simulink model "threeDiskOscillatorRig"  (R2024a)
settings: Solver=VariableStepAuto  StartTime=0.0  StopTime=SIM_TIME  RelTol=1e-8
values from neighbouring files (symbols this model uses):
  C = [0 0 0 0 1 0]    [Assignment2.m]
undefined symbols (not defined in the file or in its folder): atan_scale, b_1, b_2, b_3, J_1, J_2, J_3, k_1, k_2, Kred_tf_d, sigma1, SIM_TIME, T_Cm, T_Cp, T_s, w_th, x_0
libraries: simulink x1
settings Model: Creator=dimpa  LastModifiedBy=szica
settings SolverCC: AlgebraicLoopSolver=TrustRegion
settings DataIOCC: ReturnWorkspaceOutputs=off
settings DebuggingCC: UnconnectedInputMsg=warning  UnconnectedOutputMsg=warning  UnconnectedLineMsg=warning  ArithmeticOperatorsInVariantConditions=warning
settings ModelReferenceCC: EnableRefExpFcnMdlSchedulingChecks=on
settings SFSimCC: SimUseLocalCustomCode=off  CustomCodeUndefinedFunction=UseInterfaceOnly
settings RTWCC: RTWUseLocalCustomCode=off  GPUComputeCapability=3.5  DLArmComputeVersion=19.05

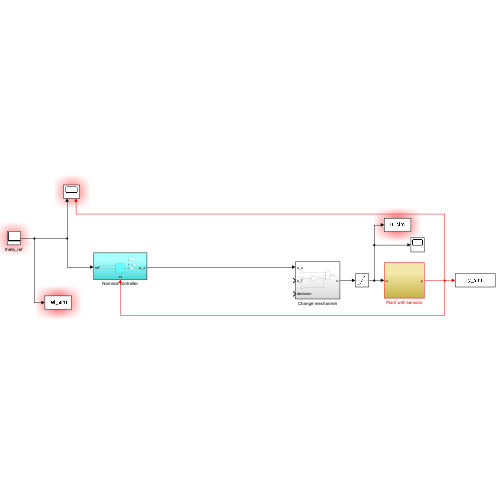
[thumbnail: Simulink's stored preview of the top-level diagram]
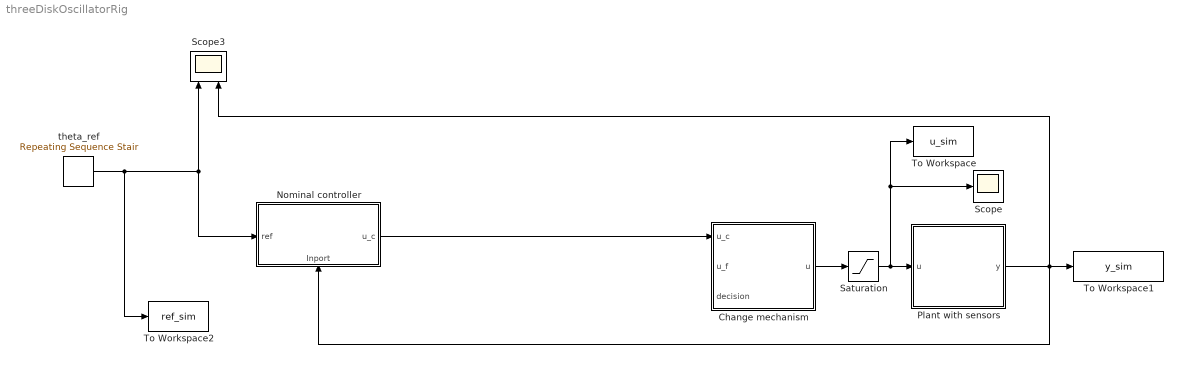
== system threeDiskOscillatorRig ==
  Change mechanism : Subsystem
  Nominal controller : Subsystem
      settings: PortSchema="{\"entries\":[{\"content\":{\"sides\":[{\"content\":{\"connectorIds\":[\"In1\"]},\"type\":\"ConnectorPlacement.EquallySpacedRectSide\",\"uuid\":\"4a12b61f-9c5c-4b70-9adc-3d80c48385d1\"},{\"content\":{\"connectorIds\":[\"Out1\"],\"side\":\"RIGHT\"},\"type\":\"ConnectorPlacement.EquallySpacedRectSide\",\"uuid\":\"2083013e-02ec-4e33-92aa-a5e5c42c1a52\"},{\"content\":{\"side\":\"TOP\"},\"type\":\"ConnectorPlacement.EquallySpacedRectSide\",\"uuid\":\"64789157-88d0-4aa4-87ae-72576a40396a\"},{\"content\":{\"connectorIds\":[\"In2\"],\"side\":\"BOTTOM\"},\"type\":\"ConnectorPlacement.EquallySpacedRectSide\",\"uuid\":\"628a79db-f9b2-407d-a20c-25144858a4c1\"}]},\"type\":\"ConnectorPlacement.EquallySpacedConnector\",\"uuid\":\"5f7ce1a9-4de3-49cc-b1cc-2f956a8eb5ad\"}],\"packageUris\":[\"http://schema.mathworks.com/mf0/Connector/R2020b\"],\"version\":\"1.0\"}"
  Plant with sensors : Subsystem
  Saturation : Saturate  UpperLimit=2  LowerLimit=-2
  Scope : Scope
  Scope3 : Scope  NumInputPorts=2
  To Workspace : ToWorkspace  VariableName=u_sim  SaveFormat=Timeseries  SampleTime=T_s
  To Workspace1 : ToWorkspace  VariableName=y_sim  SaveFormat=Timeseries  SampleTime=-1
  To Workspace2 : ToWorkspace  VariableName=ref_sim  SaveFormat=Timeseries  SampleTime=T_s
  theta_ref : simulink/Sources/Repeating Sequence Stair  OutValues=[0 0 0]  tsamp=SIM_TIME/2  OutMin=[]  OutMax=[]  OutDataTypeStr=double  OutputDataTypeScalingMode=double  OutDataType=fixdt(0,8)  ConRadixGroup=Best Precision: Vector-wise  OutScaling=2^-12
  wires:
  Plant with sensors/1(y) -> To Workspace1/1, Scope3/2, Nominal controller/2(Inport)
  theta_ref/1 -> Nominal controller/1(ref), Scope3/1, To Workspace2/1
  Change mechanism/1(u) -> Saturation/1
  Nominal controller/1(u_c) -> Change mechanism/1(u_c)
  Saturation/1 -> To Workspace/1, Scope/1, Plant with sensors/1(u)

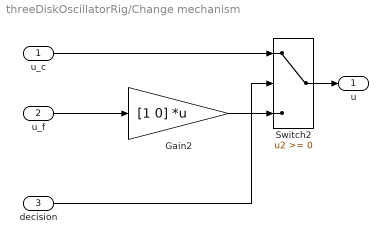
== system threeDiskOscillatorRig/Change mechanism ==
  u_c : Inport
  u_f : Inport  Port=2
  decision : Inport  Port=3
  Gain2 : Gain  Gain=[1 0]  Multiplication=Matrix(K*u) (u vector)
  Switch2 : Switch  OutDataTypeStr=double  SaturateOnIntegerOverflow=off  InputSameDT=off
  u : Outport
  wires:
  Gain2/1 -> Switch2/3
  decision/1 -> Switch2/2
  u_c/1 -> Switch2/1
  Switch2/1 -> u/1
  u_f/1 -> Gain2/1

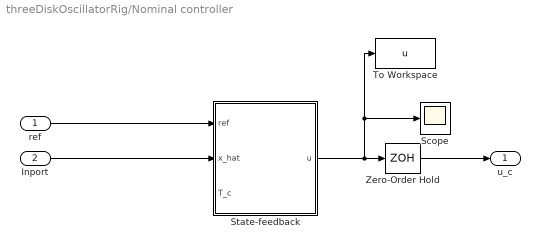
== system threeDiskOscillatorRig/Nominal controller ==
  ref : Inport
  Inport : Inport  Port=2
  Scope : Scope
  State-feedback : Subsystem
  To Workspace : ToWorkspace  VariableName=u  SaveFormat=Timeseries  SampleTime=T_s
  Zero-Order Hold : ZeroOrderHold  SampleTime=T_s
  u_c : Outport
  wires:
  Zero-Order Hold/1 -> u_c/1
  ref/1 -> State-feedback/1(ref)
  State-feedback/1(u) -> To Workspace/1, Scope/1, Zero-Order Hold/1
  Inport/1 -> State-feedback/2(x_hat)

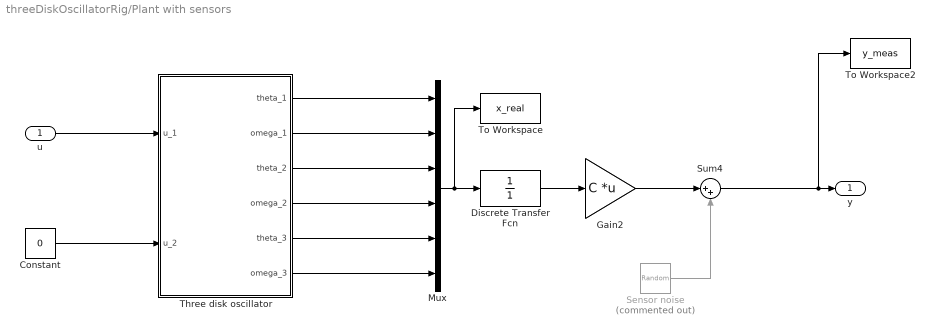
== system threeDiskOscillatorRig/Plant with sensors ==
  u : Inport
  Constant : Constant  Value=0
  Discrete Transfer Fcn : DiscreteTransferFcn  Denominator=[1]  SampleTime=T_s
  Gain2 : Gain  Gain=C  Multiplication=Matrix(K*u) (u vector)
  Mux : Mux  Inputs=6
  Sensor noise : RandomNumber  Commented=on  Variance=sigma1  SampleTime=T_s
  Sum4 : Sum  Inputs=|++
  Three disk oscillator : Subsystem
  To Workspace : ToWorkspace  VariableName=x_real  SaveFormat=Timeseries  SampleTime=T_s
  To Workspace2 : ToWorkspace  VariableName=y_meas  SaveFormat=Timeseries  SampleTime=T_s
  y : Outport  VectorParamsAs1DForOutWhenUnconnected=off
  wires:
  Three disk oscillator/2(omega_1) -> Mux/2
  Three disk oscillator/1(theta_1) -> Mux/1
  Mux/1 -> To Workspace/1, Discrete Transfer Fcn/1
  Three disk oscillator/4(omega_2) -> Mux/4
  Three disk oscillator/3(theta_2) -> Mux/3
  Discrete Transfer Fcn/1 -> Gain2/1
  Gain2/1 -> Sum4/1
  Sensor noise/1 -> Sum4/2
  Three disk oscillator/6(omega_3) -> Mux/6
  Three disk oscillator/5(theta_3) -> Mux/5
  Sum4/1 -> To Workspace2/1, y/1
  u/1 -> Three disk oscillator/1(u_1)
  Constant/1 -> Three disk oscillator/2(u_2)

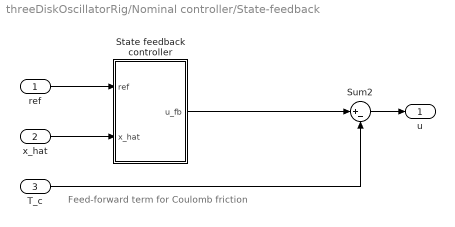
== system threeDiskOscillatorRig/Nominal controller/State-feedback ==
  note: Feed-forward term for Coulomb friction
  ref : Inport
  x_hat : Inport  Port=2
  T_c : Inport  Port=3
  State feedback controller : Subsystem
  Sum2 : Sum  Inputs=|+-
  u : Outport  VectorParamsAs1DForOutWhenUnconnected=off
  wires:
  T_c/1 -> Sum2/2
  Sum2/1 -> u/1
  ref/1 -> State feedback controller/1(ref)
  x_hat/1 -> State feedback controller/2(x_hat)
  State feedback controller/1(u_fb) -> Sum2/1

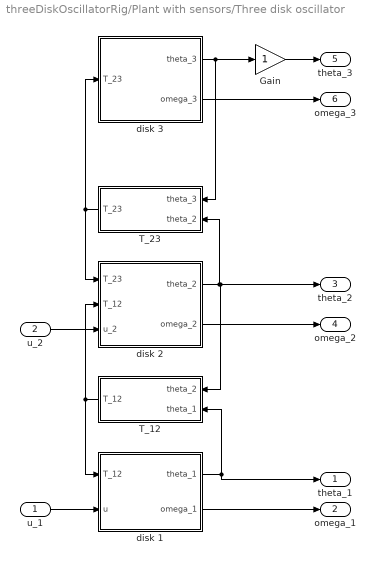
== system threeDiskOscillatorRig/Plant with sensors/Three disk oscillator ==
  u_1 : Inport
  u_2 : Inport  Port=2
  Gain : Gain
  T_12 : Subsystem
  T_23 : Subsystem
  disk 1 : Subsystem
  disk 2 : Subsystem
  disk 3 : Subsystem
  theta_1 : Outport  VectorParamsAs1DForOutWhenUnconnected=off
  omega_1 : Outport  Port=2  VectorParamsAs1DForOutWhenUnconnected=off
  theta_2 : Outport  Port=3  VectorParamsAs1DForOutWhenUnconnected=off
  omega_2 : Outport  Port=4  VectorParamsAs1DForOutWhenUnconnected=off
  theta_3 : Outport  Port=5  VectorParamsAs1DForOutWhenUnconnected=off
  omega_3 : Outport  Port=6  VectorParamsAs1DForOutWhenUnconnected=off
  wires:
  T_23/1(T_23) -> disk 2/1(T_23), disk 3/1(T_23)
  disk 1/1(theta_1) -> theta_1/1, T_12/2(theta_1)
  disk 2/1(theta_2) -> T_23/2(theta_2), theta_2/1, T_12/1(theta_2)
  T_12/1(T_12) -> disk 1/1(T_12), disk 2/2(T_12)
  disk 3/2(omega_3) -> omega_3/1
  disk 1/2(omega_1) -> omega_1/1
  disk 2/2(omega_2) -> omega_2/1
  u_1/1 -> disk 1/2(u)
  disk 3/1(theta_3) -> Gain/1, T_23/1(theta_3)
  Gain/1 -> theta_3/1
  u_2/1 -> disk 2/3(u_2)

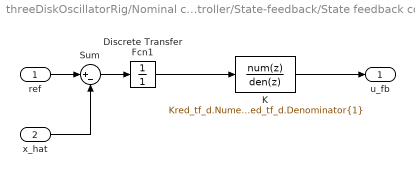
== system threeDiskOscillatorRig/Nominal controller/State-feedback/State feedback controller ==
  ref : Inport
  x_hat : Inport  Port=2
  Discrete Transfer Fcn1 : DiscreteTransferFcn  Numerator=1  Denominator=1
  K : DiscreteTransferFcn  Numerator=Kred_tf_d.Numerator{1}  Denominator=Kred_tf_d.Denominator{1}
  Sum : Sum  Inputs=|+-
  u_fb : Outport
  wires:
  Discrete Transfer Fcn1/1 -> K/1
  K/1 -> u_fb/1
  ref/1 -> Sum/1
  Sum/1 -> Discrete Transfer Fcn1/1
  x_hat/1 -> Sum/2

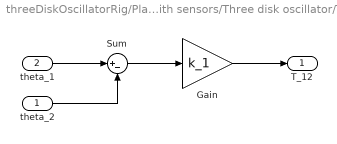
== system threeDiskOscillatorRig/Plant with sensors/Three disk oscillator/T_12 ==
  theta_2 : Inport
  theta_1 : Inport  Port=2
  Gain : Gain  Gain=k_1
  Sum : Sum  Inputs=|+-
  T_12 : Outport  VectorParamsAs1DForOutWhenUnconnected=off
  wires:
  theta_2/1 -> Sum/2
  theta_1/1 -> Sum/1
  Sum/1 -> Gain/1
  Gain/1 -> T_12/1

== system threeDiskOscillatorRig/Plant with sensors/Three disk oscillator/T_23 ==
  theta_3 : Inport
  theta_2 : Inport  Port=2
  Gain : Gain  Gain=k_2
  Sum : Sum  Inputs=-+|
  T_23 : Outport  VectorParamsAs1DForOutWhenUnconnected=off
  wires:
  Gain/1 -> T_23/1
  Sum/1 -> Gain/1
  theta_3/1 -> Sum/1
  theta_2/1 -> Sum/2

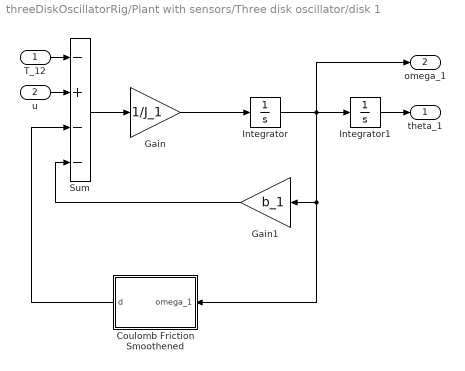
== system threeDiskOscillatorRig/Plant with sensors/Three disk oscillator/disk 1 ==
  T_12 : Inport
  u : Inport  Port=2
  Coulomb Friction Smoothened : Subsystem
  Gain : Gain  Gain=1/J_1
  Gain1 : Gain  Gain=b_1
  Integrator : Integrator  InitialCondition=x_0(2)
  Integrator1 : Integrator  InitialCondition=x_0(1)
  Sum : Sum  Inputs=-+--
  theta_1 : Outport  VectorParamsAs1DForOutWhenUnconnected=off
  omega_1 : Outport  Port=2  VectorParamsAs1DForOutWhenUnconnected=off
  wires:
  Sum/1 -> Gain/1
  Integrator/1 -> Integrator1/1, omega_1/1, Coulomb Friction Smoothened/1(omega_1), Gain1/1
  Gain1/1 -> Sum/4
  Integrator1/1 -> theta_1/1
  T_12/1 -> Sum/1
  u/1 -> Sum/2
  Gain/1 -> Integrator/1
  Coulomb Friction Smoothened/1(d) -> Sum/3

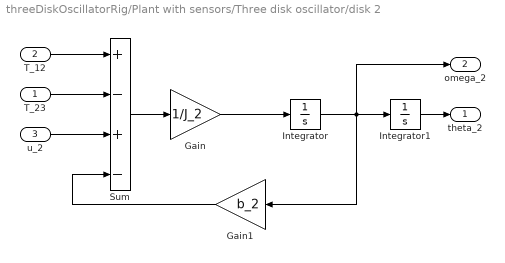
== system threeDiskOscillatorRig/Plant with sensors/Three disk oscillator/disk 2 ==
  T_23 : Inport
  T_12 : Inport  Port=2
  u_2 : Inport  Port=3
  Gain : Gain  Gain=1/J_2
  Gain1 : Gain  Gain=b_2
  Integrator : Integrator  InitialCondition=x_0(4)
  Integrator1 : Integrator  InitialCondition=x_0(3)
  Sum : Sum  Inputs=+-+-
  theta_2 : Outport  VectorParamsAs1DForOutWhenUnconnected=off
  omega_2 : Outport  Port=2  VectorParamsAs1DForOutWhenUnconnected=off
  wires:
  T_23/1 -> Sum/2
  T_12/1 -> Sum/1
  Integrator1/1 -> theta_2/1
  Gain1/1 -> Sum/4
  Gain/1 -> Integrator/1
  Integrator/1 -> Integrator1/1, Gain1/1, omega_2/1
  Sum/1 -> Gain/1
  u_2/1 -> Sum/3

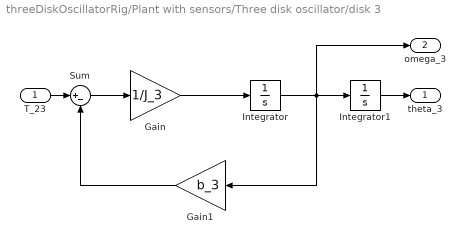
== system threeDiskOscillatorRig/Plant with sensors/Three disk oscillator/disk 3 ==
  T_23 : Inport
  Gain : Gain  Gain=1/J_3
  Gain1 : Gain  Gain=b_3
  Integrator : Integrator  InitialCondition=x_0(6)
  Integrator1 : Integrator  InitialCondition=x_0(5)
  Sum : Sum  Inputs=|+-
  theta_3 : Outport  VectorParamsAs1DForOutWhenUnconnected=off
  omega_3 : Outport  Port=2  VectorParamsAs1DForOutWhenUnconnected=off
  wires:
  Sum/1 -> Gain/1
  Integrator/1 -> Integrator1/1, omega_3/1, Gain1/1
  Gain/1 -> Integrator/1
  Gain1/1 -> Sum/2
  Integrator1/1 -> theta_3/1
  T_23/1 -> Sum/1

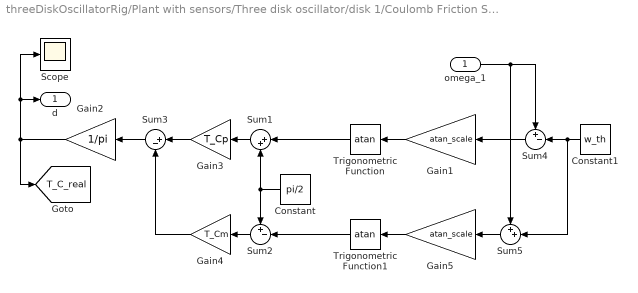
== system threeDiskOscillatorRig/Plant with sensors/Three disk oscillator/disk 1/Coulomb Friction Smoothened ==
  omega_1 : Inport
  Constant : Constant  Value=pi/2
  Constant1 : Constant  Value=w_th
  Gain1 : Gain  Gain=atan_scale
  Gain2 : Gain  Gain=1/pi
  Gain3 : Gain  Gain=T_Cp
  Gain4 : Gain  Gain=T_Cm
  Gain5 : Gain  Gain=atan_scale
  Scope : Scope
  Sum1 : Sum  Inputs=|++
  Sum2 : Sum  Inputs=+-|
  Sum3 : Sum  Inputs=|+-
  Sum4 : Sum  Inputs=+-|
  Sum5 : Sum  Inputs=++|
  Trigonometric Function : Trigonometry  Operator=atan
  Trigonometric Function1 : Trigonometry  Operator=atan
  d : Outport  VectorParamsAs1DForOutWhenUnconnected=off
  tag scope: T_C_real=global
  wires:
  Gain1/1 -> Trigonometric Function/1
  Sum1/1 -> Gain3/1
  Constant/1 -> Sum2/1, Sum1/2
  Sum2/1 -> Gain4/1
  Sum3/1 -> Gain2/1
  Trigonometric Function/1 -> Sum1/1
  Gain4/1 -> Sum3/2
  Gain2/1 -> [T_C_real], Scope/1, d/1
  omega_1/1 -> Sum5/1, Sum4/1
  Gain3/1 -> Sum3/1
  Sum4/1 -> Gain1/1
  Constant1/1 -> Sum5/2, Sum4/2
  Gain5/1 -> Trigonometric Function1/1
  Sum5/1 -> Gain5/1
  Trigonometric Function1/1 -> Sum2/2
